simulink model "modelo_mma"  (R2015a)
settings: Solver=ode45  StartTime=0.0  StopTime=50  RelTol=1e-6  AbsTol=1e-6
values from neighbouring files (symbols this model uses):
  B = 1e-1    (= 0.1)    [var_mma.m]
  k = 1    [var_mma.m]
  m = 1    [var_mma.m]
libraries: fl_lib x7, nesl_utility x3
settings Model: Creator=11802972  LastModifiedBy=11802972

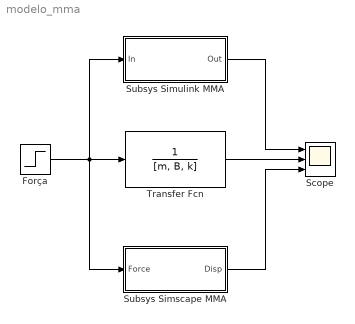
== system modelo_mma ==
  Força : Step  After=10  SampleTime=0
  Scope : Scope  NumInputPorts=3
      settings: YMin=-5~-5~-5  YMax=5~5~5
  Subsys Simscape MMA : Subsystem
  Subsys Simulink MMA : Subsystem
  Transfer Fcn : TransferFcn  Denominator=[m, B, k]
  wires:
  Força/1 -> Subsys Simscape MMA/1(Force), Subsys Simulink MMA/1(In), Transfer Fcn/1
  Subsys Simulink MMA/1(Out) -> Scope/1
  Transfer Fcn/1 -> Scope/2
  Subsys Simscape MMA/1(Disp) -> Scope/3

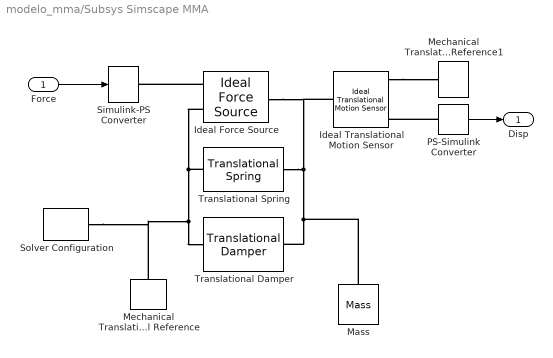
== system modelo_mma/Subsys Simscape MMA ==
  Force : Inport
  Ideal Force Source : fl_lib/Mechanical/Mechanical Sources/Ideal Force Source
  Ideal Translational Motion Sensor : fl_lib/Mechanical/Mechanical Sensors/Ideal Translational Motion Sensor  offset=0 m
  Mass : fl_lib/Mechanical/Translational Elements/Mass  mass=m kg  v_specify=off  v_priority=High  v=0 m/s  f_specify=off  f_priority=High  f=0 N
  Mechanical Translational Reference : fl_lib/Mechanical/Translational Elements/Mechanical Translational Reference
  Mechanical Translational Reference1 : fl_lib/Mechanical/Translational Elements/Mechanical Translational Reference
  PS-Simulink Converter : nesl_utility/PS-Simulink Converter  PhysicalDomain=network_engine_domain  SubClassName=ps_output  LeftPortType=input  RightPortType=output  PseudoPeriodic=off  Frequencies=[]  Unit=1  AffineConversion=off
  Simulink-PS Converter : nesl_utility/Simulink-PS Converter  PhysicalDomain=network_engine_domain  SubClassName=ps_input  LeftPortType=input  RightPortType=output  PseudoPeriodic=off  Frequencies=[]  NoiseDistribution=none  NoiseParameters=[]  Unit=1  AffineConversion=off  InputFiltering=off  SimscapeFilterOrder=1  InputFilterTimeConstant=0.001  UdotUserProvided=1
  Solver Configuration : nesl_utility/Solver Configuration  PhysicalDomain=network_engine_domain  SubClassName=solver  LeftPortType=input  RightPortType=generic  Accelerate=off  Tones=[]  Harmonics=[]  SimulateNoise=off  Profile=off  UseLocalSampling=off  EnableSwitchedLinearOptims=on  FrequencyDomain=off  UseCCode=off  RelTol=0.001  AbsTol=1e-06  MinStep=1e-09  ToWorkspace=off  RevertToSquareIcSolve=off  NumHomotopyIterations=100  DoDC=off  ResidualTolerance=1e-09  UseLocalSolver=off  LocalSolverChoice=NE_BACKWARD_EULER_ADVANCER  LocalSolverSampleTime=0.001  DoFixedCost=off  MaxNonlinIter=3  MaxModeIter=2  LinearAlgebra=Sparse  DelaysMemoryBudget=1024  AutomaticFiltering=on  FilteringTimeConstant=0.001
  Translational Damper : fl_lib/Mechanical/Translational Elements/Translational Damper  D=B N/(m/s)  v_specify=off  v_priority=High  v=0 m/s  f_specify=off  f_priority=High  f=0 N
  Translational Spring : fl_lib/Mechanical/Translational Elements/Translational Spring  spr_rate=k N/m  v_specify=off  v_priority=High  v=0 m/s  f_specify=off  f_priority=High  f=0 N  x_specify=off  x_priority=High  x=0 m
  Disp : Outport
  wires:
  Force/1 -> Simulink-PS Converter/1
  PS-Simulink Converter/1 -> Disp/1
  connections:
  Translational Spring/LConn1 -- Solver Configuration/RConn1 -- Mechanical Translational Reference/LConn1 -- Translational Damper/LConn1 -- Ideal Force Source/RConn2
  Translational Spring/RConn1 -- Mass/LConn1 -- Translational Damper/RConn1 -- Ideal Translational Motion Sensor/LConn1 -- Ideal Force Source/LConn1
  Ideal Force Source/RConn1 -- Simulink-PS Converter/RConn1
  PS-Simulink Converter/LConn1 -- Ideal Translational Motion Sensor/RConn3
  Ideal Translational Motion Sensor/RConn1 -- Mechanical Translational Reference1/LConn1

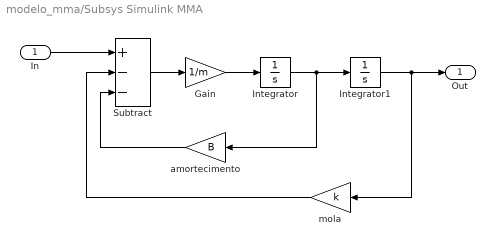
== system modelo_mma/Subsys Simulink MMA ==
  In : Inport
  Gain : Gain  Gain=1/m
  Integrator : Integrator
  Integrator1 : Integrator
  Subtract : Sum  Inputs=+--
  amortecimento : Gain  Gain=B
  mola : Gain  Gain=k
  Out : Outport
  wires:
  In/1 -> Subtract/1
  Subtract/1 -> Gain/1
  Gain/1 -> Integrator/1
  Integrator/1 -> amortecimento/1, Integrator1/1
  amortecimento/1 -> Subtract/3
  mola/1 -> Subtract/2
  Integrator1/1 -> Out/1, mola/1
